simulink model "square_wave_generator"  (R2023a)
settings: Solver=VariableStepAuto  StartTime=0.0  StopTime=10.0  RelTol=1e-3
values from neighbouring files (symbols this model uses):
  wave_amplitude = deg2rad(15)    [ELEN90064_Project_Parameters.m]
  wave_offset = deg2rad(30)    [ELEN90064_Project_Parameters.m]
  wave_period = 6    [ELEN90064_Project_Parameters.m]
settings Model: Creator=yunzh  LastModifiedBy=yunzh

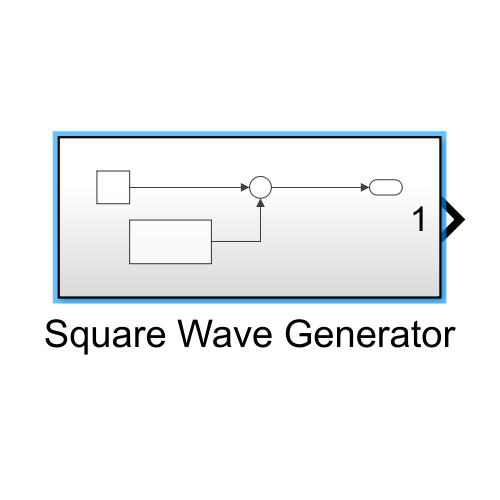
[thumbnail: Simulink's stored preview of the top-level diagram]
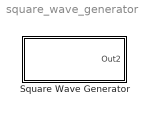
== system square_wave_generator ==
  Square Wave Generator : Subsystem

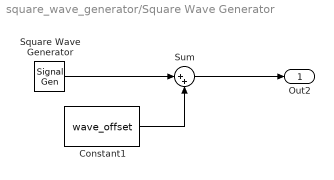
== system square_wave_generator/Square Wave Generator ==
  Constant1 : Constant  Value=wave_offset
  Square Wave Generator : SignalGenerator  WaveForm=square  Amplitude=wave_amplitude  Frequency=1 / wave_period
  Sum : Sum  Inputs=|++
  Out2 : Outport
  wires:
  Square Wave Generator/1 -> Sum/1
  Constant1/1 -> Sum/2
  Sum/1 -> Out2/1
